simulink model "H_inf_modelo"  (R2024a)
settings: Solver=VariableStepAuto  StartTime=0.0  StopTime=50  RelTol=1e-3
values from neighbouring files (symbols this model uses):
  K = K    [Proyecto_Hinf_incompleto.m]
undefined symbols (not defined in the file or in its folder): Aa, Bb, C
libraries: simulink x1
settings Model: Creator=PERSONAL  LastModifiedBy=Luis Enrique Carmona
settings RTWCC: GPUComputeCapability=3.5

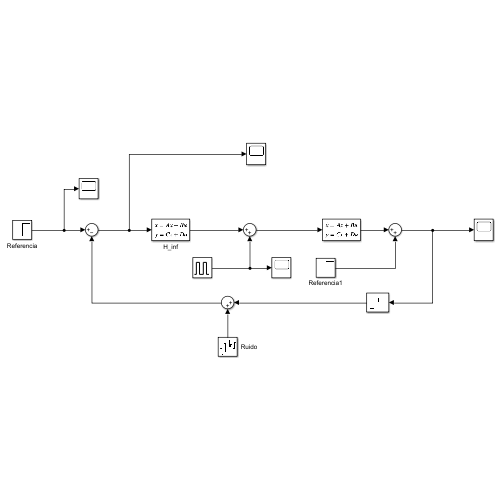
[thumbnail: Simulink's stored preview of the top-level diagram]
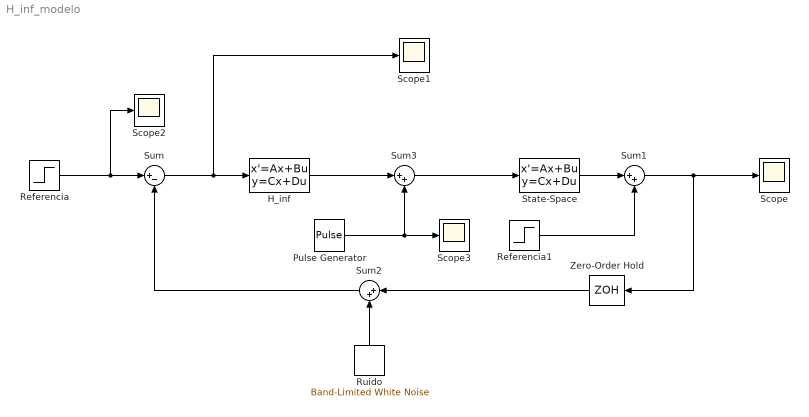
== system H_inf_modelo ==
  H_inf : StateSpace  A=K.A  B=K.B  C=K.C  D=K.D  InitialCondition=0
  Pulse Generator : DiscretePulseGenerator  PulseType=Time based  Period=22  PulseWidth=5  PhaseDelay=1
  Referencia : Step  Time=0  After=50  SampleTime=0
  Referencia1 : Step  Time=0  After=50  SampleTime=0
  Ruido : simulink/Sources/Band-Limited White Noise  Cov=[1]  Ts=0.1  seed=[23341]
  Scope{,1..3} (4 alike) : Scope
  State-Space : StateSpace  A=Aa  B=Bb  C=C  D=0  InitialCondition=-20
  Sum : Sum  Inputs=|+-
  Sum1 : Sum  Inputs=|++
  Sum2 : Sum  Inputs=|++
  Sum3 : Sum  Inputs=|++
  Zero-Order Hold : ZeroOrderHold  SampleTime=0.01
  wires:
  Referencia/1 -> Scope2/1, Sum/1
  Sum/1 -> Scope1/1, H_inf/1
  H_inf/1 -> Sum3/1
  Sum2/1 -> Sum/2
  Sum3/1 -> State-Space/1
  Pulse Generator/1 -> Sum3/2, Scope3/1
  Zero-Order Hold/1 -> Sum2/1
  State-Space/1 -> Sum1/1
  Sum1/1 -> Zero-Order Hold/1, Scope/1
  Referencia1/1 -> Sum1/2
  Ruido/1 -> Sum2/2
